simulink model "thermostat_task"  (Simulink 3.00)
libraries: mathlib x3, arclib x2, analoglib x1, logiclib x1

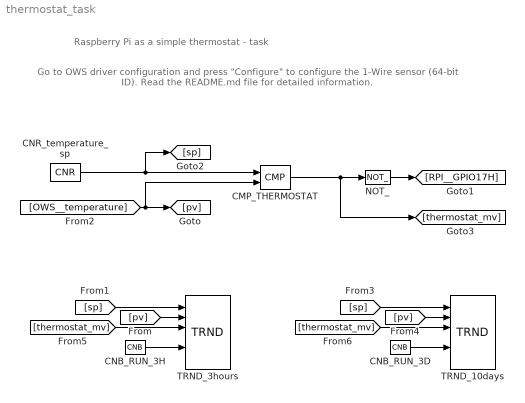
== system thermostat_task ==
  note: Go to OWS driver configuration and press "Configure" to configure the 1-Wire sensor (64-bit ID).
      |
      | Read the README.md file for detailed information.
  note: Raspberry Pi as a simple thermostat - task
  CMP_THERMOSTAT : analoglib/CMP  hys=0.5
  CNB_RUN_3D : mathlib/CNB  YCN=on
  CNB_RUN_3H : mathlib/CNB  YCN=on
  CNR_temperature_sp : mathlib/CNR  ycn=21.8
  NOT_ : logiclib/NOT_
  TRND_10days : arclib/TRND  n=4  l=86400  btype=8: Double  ptype1=1: Store  ptype2=1: Store  ptype3=1: Store  ptype4=1: Store  pfac=20  afac=0  arc=0  id=1  Title=Thermostat actions (10 days)  timesrc=1
  TRND_3hours : arclib/TRND  n=4  l=10800  btype=8: Double  ptype1=1: Store  ptype2=1: Store  ptype3=1: Store  ptype4=1: Store  pfac=2  afac=0  arc=0  id=1  Title=Thermostat actions (3 hours)  timesrc=1
  wires:
  CMP_THERMOSTAT/1 -> [thermostat_mv], NOT_/1
  CNB_RUN_3D/1 -> TRND_10days/5
  CNB_RUN_3H/1 -> TRND_3hours/5
  CNR_temperature_sp/1 -> CMP_THERMOSTAT/1, [sp]
  [pv] -> TRND_3hours/2
  [sp] -> TRND_3hours/1
  [OWS__temperature] -> CMP_THERMOSTAT/2, [pv]
  [sp] -> TRND_10days/1
  [pv] -> TRND_10days/2
  [thermostat_mv] -> TRND_3hours/3
  [thermostat_mv] -> TRND_10days/3
  NOT_/1 -> [RPI__GPIO17H]
